simulink model "TestFuncionality"  (Simulink 7.4)
settings: Solver=FixedStepDiscrete  StartTime=0.0  StopTime=10.0  FixedStep=1  RelTol=1e-3
libraries: MPCMdlLib x25
settings Model: Creator=serg  LastModifiedBy=Serg
settings OptimizationCC: InitFltsAndDblsToZero=on

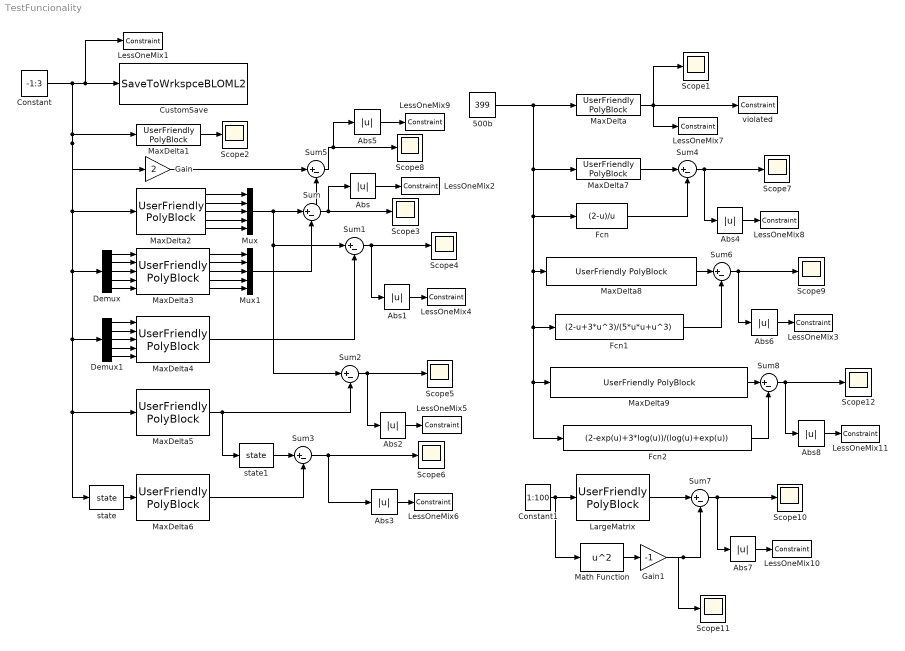
== system TestFuncionality ==
  500b : Constant  Value=399  OutDataType=sfix(16)  OutScaling=2^0
  Abs{,1..8} (9 alike) : Abs  OutDataType=sfix(16)  OutScaling=2^0
  Constant : Constant  Value=-1:3  OutDataType=sfix(16)  OutScaling=2^0
  Constant1 : Constant  Value=1:100  OutDataType=sfix(16)  OutScaling=2^0
  CustomSave : M-S-Function  FunctionName=SaveToWrkspceBLOML2  Parameters='srg'
  Demux : Demux  Outputs=5
  Demux1 : Demux  Outputs=5
  Fcn : Fcn  Expr=(2-u)/u
  Fcn1 : Fcn  Expr=(2-u+3*u^3)/(5*u*u+u^3)
  Fcn2 : Fcn  Expr=(2-exp(u)+3*log(u))/(log(u)+exp(u))
  Gain : Gain  Gain=2  ParameterDataType=sfix(16)  ParameterScaling=2^0  OutDataType=sfix(16)  OutScaling=2^0
  Gain1 : Gain  Gain=-1  ParameterDataType=sfix(16)  ParameterScaling=2^0  OutDataType=sfix(16)  OutScaling=2^0
  LargeMatrix : MPCMdlLib/UserFriendly PolyBlock  Tag=PolyBlock  A=eye(100)*2  C=eye(100)  gA=zeros(1,100)  gC=-1  input_type=Vector  output_type=Vector  port_names=u
  LessOneMix1 : MPCMdlLib/Constraint  Tag=InequalBlock  CompareSign=> 0
  LessOneMix{2..11} (10 alike) : MPCMdlLib/Constraint  Tag=InequalBlock  CompareSign=< 0
  Math Function : Math  Operator=square  OutDataType=sfix(16)  OutScaling=2^0  SaturateOnIntegerOverflow=on
  MaxDelta : MPCMdlLib/UserFriendly PolyBlock  Tag=PolyBlock  A="[0  ;1]"  C=[2 -1]  gA=[0 ]  gC=1  input_type=Scalar  output_type=Scalar  port_names=u
  MaxDelta1 : MPCMdlLib/UserFriendly PolyBlock  Tag=PolyBlock  A=eye(5)  C=[1:5]  gA=zeros(1,5)  gC=1  input_type=Vector  output_type=Scalar  port_names=u
  MaxDelta2 : MPCMdlLib/UserFriendly PolyBlock  Tag=PolyBlock  A=eye(5)  C=2*eye(5)  gA=zeros(1,5)  gC=1  input_type=Vector  output_type=Scalar  port_names=u
  MaxDelta3 : MPCMdlLib/UserFriendly PolyBlock  Tag=PolyBlock  A=eye(5)  C=2*eye(5)  gA=zeros(1,5)  gC=1  input_type=Scalar  output_type=Scalar  port_names=u
  MaxDelta4 : MPCMdlLib/UserFriendly PolyBlock  Tag=PolyBlock  A=eye(5)  C=2*eye(5)  gA=zeros(1,5)  gC=1  input_type=Scalar  output_type=Vector  port_names=u
  MaxDelta5 : MPCMdlLib/UserFriendly PolyBlock  Tag=PolyBlock  A=eye(5)  C=2*eye(5)  gA=zeros(1,5)  gC=1  input_type=Vector  output_type=Vector  port_names=u
  MaxDelta6 : MPCMdlLib/UserFriendly PolyBlock  Tag=PolyBlock  A=eye(5)  C=2*eye(5)  gA=zeros(1,5)  gC=1  input_type=Vector  output_type=Vector  port_names=u
  MaxDelta7 : MPCMdlLib/UserFriendly PolyBlock  Tag=PolyBlock  A="[0  ;1]"  C=[2 -1]  gA=[1 ]  gC=1  input_type=Scalar  output_type=Scalar  port_names=u
  MaxDelta8 : MPCMdlLib/UserFriendly PolyBlock  Tag=PolyBlock  A="[0  ;1 ; 3]"  C=[2 -1 3]  gA=[2; 3]  gC=[5 1]  input_type=Scalar  output_type=Scalar  port_names=u
  MaxDelta9 : MPCMdlLib/UserFriendly PolyBlock  Tag=PolyBlock  A="[0  ;inf ; -inf]"  C=[2 -1 3]  gA=[-inf; inf]  gC=[1 1]  input_type=Scalar  output_type=Scalar  port_names=u
  Mux : Mux  Inputs=5
  Mux1 : Mux  Inputs=5
  Scope{1..12} (12 alike) : Scope
      Scope1 settings: TimeRange=10
      Scope10 settings: TimeRange=10  SaveName=ScopeData9
      Scope11 settings: TimeRange=10  SaveName=ScopeData10
      Scope12 settings: TimeRange=10  SaveName=ScopeData11
      Scope2 settings: TimeRange=10
      Scope3 settings: TimeRange=10  SaveName=ScopeData2
      Scope4 settings: TimeRange=10  SaveName=ScopeData3
      Scope5 settings: TimeRange=10  SaveName=ScopeData4
      Scope6 settings: TimeRange=10  SaveName=ScopeData5
      Scope7 settings: TimeRange=10  SaveName=ScopeData6
      Scope8 settings: TimeRange=10  SaveName=ScopeData7
      Scope9 settings: TimeRange=10  SaveName=ScopeData8
  Sum{,1..8} (9 alike) : Sum  Inputs=|+-  OutDataType=sfix(16)  OutScaling=2^0
  state : MPCMdlLib/state  Tag=OptState  SystemSampleTime=-1  init_val=0  save_name=BL_state
  state1 : MPCMdlLib/state  Tag=OptState  SystemSampleTime=-1  init_val=0  save_name=BL_state1
  violated : MPCMdlLib/Constraint  Tag=InequalBlock  CompareSign=> 0
  wires:
  Constant/1 -> CustomSave/1, LessOneMix1/1, MaxDelta1/1, MaxDelta2/1, Demux/1, Demux1/1, state/1, MaxDelta5/1, Gain/1
  MaxDelta/1 -> violated/1, Scope1/1, LessOneMix7/1
  500b/1 -> MaxDelta/1, MaxDelta7/1, Fcn/1, MaxDelta8/1, Fcn1/1, MaxDelta9/1, Fcn2/1
  MaxDelta1/1 -> Scope2/1
  Demux/1 -> MaxDelta3/1
  Demux/2 -> MaxDelta3/2
  Demux/3 -> MaxDelta3/3
  Demux/4 -> MaxDelta3/4
  Demux/5 -> MaxDelta3/5
  Demux1/1 -> MaxDelta4/1
  Demux1/2 -> MaxDelta4/2
  Demux1/3 -> MaxDelta4/3
  Demux1/4 -> MaxDelta4/4
  Demux1/5 -> MaxDelta4/5
  MaxDelta2/1 -> Mux/1
  MaxDelta2/2 -> Mux/2
  MaxDelta2/3 -> Mux/3
  MaxDelta2/4 -> Mux/4
  MaxDelta2/5 -> Mux/5
  MaxDelta3/1 -> Mux1/1
  MaxDelta3/2 -> Mux1/2
  MaxDelta3/3 -> Mux1/3
  MaxDelta3/4 -> Mux1/4
  MaxDelta3/5 -> Mux1/5
  Mux/1 -> Sum/1, Sum1/1, Sum2/1, Sum5/2
  Mux1/1 -> Sum/2
  MaxDelta4/1 -> Sum1/2
  Sum/1 -> Scope3/1, Abs/1
  Sum1/1 -> Scope4/1, Abs1/1
  Abs/1 -> LessOneMix2/1
  Abs1/1 -> LessOneMix4/1
  Sum2/1 -> Abs2/1, Scope5/1
  Abs2/1 -> LessOneMix5/1
  MaxDelta5/1 -> Sum2/2, state1/1
  state/1 -> MaxDelta6/1
  MaxDelta6/1 -> Sum3/2
  Sum3/1 -> Abs3/1, Scope6/1
  Abs3/1 -> LessOneMix6/1
  state1/1 -> Sum3/1
  Sum4/1 -> Abs4/1, Scope7/1
  Abs4/1 -> LessOneMix8/1
  MaxDelta7/1 -> Sum4/1
  Fcn/1 -> Sum4/2
  Constant1/1 -> LargeMatrix/1, Math Function/1
  Sum5/1 -> Abs5/1, Scope8/1
  Abs5/1 -> LessOneMix9/1
  Sum6/1 -> Scope9/1, Abs6/1
  Abs6/1 -> LessOneMix3/1
  MaxDelta8/1 -> Sum6/1
  Fcn1/1 -> Sum6/2
  Gain/1 -> Sum5/1
  Sum7/1 -> Abs7/1, Scope10/1
  Abs7/1 -> LessOneMix10/1
  LargeMatrix/1 -> Sum7/1
  Math Function/1 -> Gain1/1
  Gain1/1 -> Sum7/2, Scope11/1
  Sum8/1 -> Scope12/1, Abs8/1
  Abs8/1 -> LessOneMix11/1
  Fcn2/1 -> Sum8/2
  MaxDelta9/1 -> Sum8/1
